simulink model "Host_handson"  (R2017a)
settings: Solver=FixedStepAuto  StartTime=0.0  StopTime=inf  RelTol=1e-3  EnableMultiTasking=on
libraries: c2000scilib x2, demo_controls x1
settings Model: Creator=aancelle  LastModifiedBy=ata.otaran
settings DataIOCC: LimitDataPoints=on  SaveFormat=Array  SignalLoggingSaveFormat=ModelDataLogs
settings OptimizationCC: BlockReduction=off  LifeSpan=1
settings DebuggingCC: UnderspecifiedInitializationDetection=Classic  MergeDetectMultiDrivingBlocksExec=none  SolverPrmCheckMsg=warning  AllowSymbolicDim=off  SFUnexpectedBacktrackingDiag=warning  SFNoUnconditionalDefaultTransitionDiag=warning  SFExecutionAtInitializationDiag=none
settings HardwareCC: ProdBitPerPointer=32  ProdBitPerSizeT=32  ProdBitPerPtrDiffT=32  ProdLargestAtomicFloat=None  ProdIntDivRoundTo=Undefined  ProdEndianess=Unspecified  ProdWordSize=32  ProdHWDeviceType=32-bit Generic
settings ModelReferenceCC: PropagateSignalLabelsOutOfModel=off
settings SFSimCC: MATLABDynamicMemAlloc=off
settings RTWCC: SystemTargetFile=ert.tlc  TemplateMakefile=ert_default_tmf  Description=Real-Time Workshop Embedded Coder  GenerateReport=on  IncludeHyperlinkInReport=on  LaunchReport=on  GenerateTraceInfo=on  GenerateTraceReport=on  GenerateTraceReportSl=on  GenerateTraceReportSf=on  GenerateTraceReportEml=on
settings CodeAppCC: IgnoreCustomStorageClasses=off  InternalIdentifier=Classic
settings ERTTargetCC: MultiwordLength=2048  GenerateSampleERTMain=on  ERTCustomFileTemplate=example_file_process.tlc  ConvertIfToSwitch=off  SuppressUnreachableDefaultCases=off
settings ConfigComp: CovMetricSettings=dw  CovHtmlReporting=on  CovSaveCumulativeToWorkspaceVar=on  CovSaveSingleToWorkspaceVar=on  CovExternalEMLEnable=off

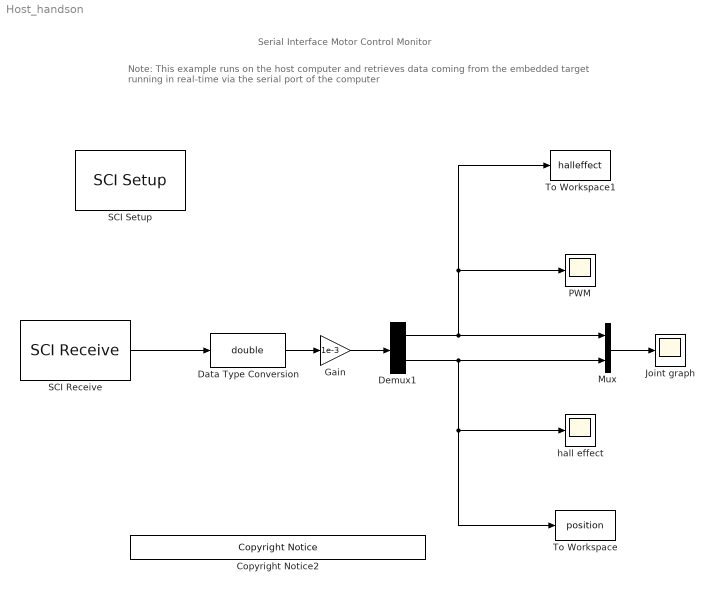
== system Host_handson ==
  note: Note: This example runs on the host computer and retrieves data
      | coming from the embedded target running in real-time via the serial port of the computer
  note: Serial Interface Motor Control Monitor
  Copyright Notice2 : demo_controls/Copyright Notice  year=2014  prod=tic2000
  Data Type Conversion : DataTypeConversion  OutDataTypeStr=double  ConvertRealWorld=Stored Integer (SI)
  Demux1 : Demux  Outputs=2
  Gain : Gain  Gain=1e-3
  Joint graph : Scope
  Mux : Mux  Inputs=2
  PWM : Scope
  SCI Receive : c2000scilib/SCI Receive  module=COM 2  dataHead='S'  dataTail='E'  dataType=int32  dataDim=2  initValue=0  errOption=Output the last received value  errValue=0  sampleTime=0.01  outputStatus=off
  SCI Setup : c2000scilib/SCI Setup  Priority=-99  commModeA=raw data  baudRateA=115200  charLenA=8  stopBitA=1  parityA=none  timeoutA=1.0  commModeB=raw data  baudRateB=115200  charLenB=8  stopBitB=1  parityB=none  timeoutB=1.0  commModeC=raw data  baudRateC=115200  charLenC=8  stopBitC=1  parityC=none  timeoutC=1.0  commModeD=raw data  baudRateD=115200  charLenD=8  stopBitD=1  parityD=none  timeoutD=1.0
  To Workspace : ToWorkspace  VariableName=position  SampleTime=-1
  To Workspace1 : ToWorkspace  VariableName=halleffect  SampleTime=-1
  hall effect : Scope
  wires:
  SCI Receive/1 -> Data Type Conversion/1
  Data Type Conversion/1 -> Gain/1
  Demux1/1 -> Mux/1, To Workspace1/1, PWM/1
  Demux1/2 -> hall effect/1, To Workspace/1, Mux/2
  Gain/1 -> Demux1/1
  Mux/1 -> Joint graph/1
